simulink model "zengiangcircle"  (Simulink 8.3)
settings: Solver=ode3  StartTime=0.0  StopTime=1500  FixedStep=0.3  RelTol=1e-3
libraries: simulink x1
settings Model: Creator=Administrator  LastModifiedBy=jackyjing
settings OptimizationCC: ExpressionDepthLimit=2147483647
settings DebuggingCC: FcnCallInpInsideContextMsg=UseLocalSettings

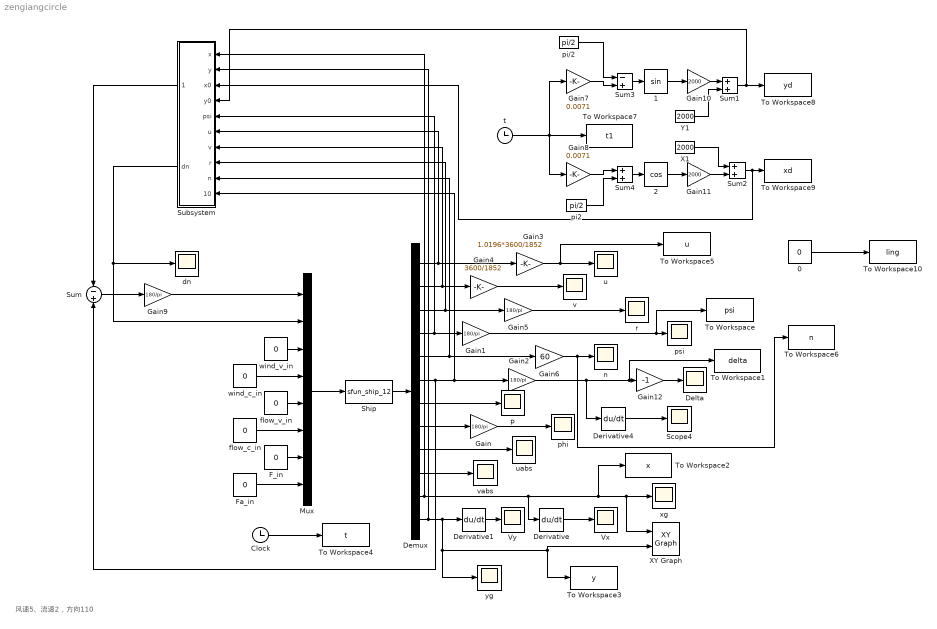
== system zengiangcircle ==
  note: 风速5、流速2，方向110
  "  1" : Trigonometry
  " 2" : Trigonometry  Operator=cos
  0 : Constant  Value=0
  Clock : Clock
  Delta : Scope
      settings: TickLabels=on  TimeRange=1500  YMin=-2  YMax=10  SaveName=ScopeData5
  Demux : Demux  Outputs=12
  Derivative : Derivative
  Derivative1 : Derivative
  Derivative4 : Derivative
  F_in : Constant  Value=0
  Fa_in : Constant  Value=0
  Gain{,1..2,5,9} (5 alike) : Gain  Gain=180/pi
  Gain10 : Gain  Gain=2000
  Gain11 : Gain  Gain=2000
  Gain12 : Gain  Gain=-1
  Gain3 : Gain  Gain=1.0196*3600/1852
  Gain4 : Gain  Gain=3600/1852
  Gain6 : Gain  Gain=60
  Gain7 : Gain  Gain=0.0071
  Gain8 : Gain  Gain=0.0071
  Mux : Mux  Inputs=8
  Scope4 : Scope
      settings: YMin=-0.005  YMax=0.002  SaveName=ScopeData18
  Ship : S-Function  FunctionName=sfun_ship_12  EnableBusSupport=off
  Subsystem : Subsystem
  Sum : Sum  Inputs=-|+
  Sum1 : Sum
  Sum2 : Sum
  Sum3 : Sum  Inputs=-+
  Sum4 : Sum
  To Workspace : ToWorkspace  VariableName=psi  SampleTime=-1
  To Workspace1 : ToWorkspace  VariableName=delta  SampleTime=-1
  To Workspace10 : ToWorkspace  VariableName=ling  SampleTime=-1
  To Workspace2 : ToWorkspace  VariableName=x  SampleTime=-1
  To Workspace3 : ToWorkspace  VariableName=y  SampleTime=-1
  To Workspace4 : ToWorkspace  VariableName=t  SampleTime=-1
  To Workspace5 : ToWorkspace  VariableName=u  SampleTime=-1
  To Workspace6 : ToWorkspace  VariableName=n  SampleTime=-1
  To Workspace7 : ToWorkspace  VariableName=t1  SampleTime=-1
  To Workspace8 : ToWorkspace  VariableName=yd  SampleTime=-1
  To Workspace9 : ToWorkspace  VariableName=xd  SampleTime=-1
  Vx : Scope
      settings: TickLabels=on  SaveName=ScopeData8
  Vy : Scope
      settings: TickLabels=on  SaveName=ScopeData9
  X1 : Constant  Value=2000
  XY Graph : simulink/Sinks/XY Graph  xmin=-1000  xmax=4500  ymin=-1000  ymax=4500  st=-1
  Y1 : Constant  Value=2000
  dn : Scope
      settings: TickLabels=on  YMin=-1.75e-05  YMax=3.75e-05  SaveName=ScopeData21
  flow_c_in : Constant  Value=0
  flow_v_in : Constant  Value=0
  n : Scope
      settings: TickLabels=on  TimeRange=1500  YMin=85.76  YMax=85.97  SaveName=ScopeData4
  p : Scope
      settings: TickLabels=on  SaveName=ScopeData10
  phi : Scope
      settings: YMin=-0.00175  YMax=0.0015  SaveName=ScopeData11
  pi/2 : Constant  Value=pi/2
  "pi2   " : Constant  Value=pi/2
  psi : Scope
      settings: TickLabels=on  TimeRange=500  YMin=-0  YMax=27.5  SaveName=ScopeData3
  r : Scope
      settings: TickLabels=on  SaveName=ScopeData2
  t : Clock
  u : Scope
      settings: TickLabels=on  YMin=25.535  YMax=25.61
  uabs : Scope
      settings: TickLabels=on  YMin=10.75  YMax=15  SaveName=ScopeData6
  v : Scope
      settings: TickLabels=on
  vabs : Scope
      settings: TickLabels=on  YMin=-1.75  YMax=0  SaveName=ScopeData7
  wind_c_in : Constant  Value=0
  wind_v_in : Constant  Value=0
  xg : Scope
      settings: TickLabels=on  YMin=250  YMax=475  SaveName=ScopeData12
  yg : Scope
      settings: TickLabels=on  YMin=250  YMax=475  SaveName=ScopeData13
  wires:
  Ship/1 -> Demux/1
  Demux/1 -> Subsystem/6(u), Gain3/1
  Demux/2 -> Subsystem/7(v), Gain4/1
  Demux/3 -> Subsystem/8(r), Gain5/1
  Demux/5 -> Subsystem/9(n), Gain6/1
  Demux/7 -> p/1
  Demux/8 -> Gain/1
  Gain1/1 -> psi/1, To Workspace/1
  Gain/1 -> phi/1
  Demux/4 -> Subsystem/5(psi), Gain1/1
  Gain3/1 -> To Workspace5/1, u/1
  Gain4/1 -> v/1
  Gain5/1 -> r/1
  Gain6/1 -> To Workspace6/1, n/1
  Demux/9 -> uabs/1
  Demux/10 -> vabs/1
  Demux/12 -> Subsystem/2(y), Derivative1/1, yg/1, To Workspace3/1, XY Graph/2
  Derivative/1 -> Vx/1
  Derivative1/1 -> Vy/1
  wind_v_in/1 -> Mux/3
  wind_c_in/1 -> Mux/4
  flow_v_in/1 -> Mux/5
  F_in/1 -> Mux/7
  Fa_in/1 -> Mux/8
  flow_c_in/1 -> Mux/6
  Mux/1 -> Ship/1
  Derivative4/1 -> Scope4/1
  Clock/1 -> To Workspace4/1
  Sum/1 -> Gain9/1
  Subsystem/1(dpsi) -> Sum/1
  Sum2/1 -> Subsystem/3(x0), To Workspace9/1
  Sum1/1 -> Subsystem/4(y0), To Workspace8/1
  "  1"/1 -> Gain10/1
  " 2"/1 -> Gain11/1
  t/1 -> To Workspace7/1, Gain8/1, Gain7/1
  Gain10/1 -> Sum1/1
  Gain11/1 -> Sum2/2
  X1/1 -> Sum2/1
  Y1/1 -> Sum1/2
  Sum3/1 -> "  1"/1
  Gain7/1 -> Sum3/2
  pi/2/1 -> Sum3/1
  Sum4/1 -> " 2"/1
  Gain8/1 -> Sum4/1
  "pi2   "/1 -> Sum4/2
  Demux/11 -> Subsystem/1(x), Derivative/1, XY Graph/1, xg/1, To Workspace2/1
  Gain9/1 -> Mux/1
  Demux/6 -> Subsystem/10(Delta), Gain2/1, Sum/2
  Subsystem/2(dn) -> dn/1, Mux/2
  0/1 -> To Workspace10/1
  Gain2/1 -> Derivative4/1, To Workspace1/1, Gain12/1
  Gain12/1 -> Delta/1

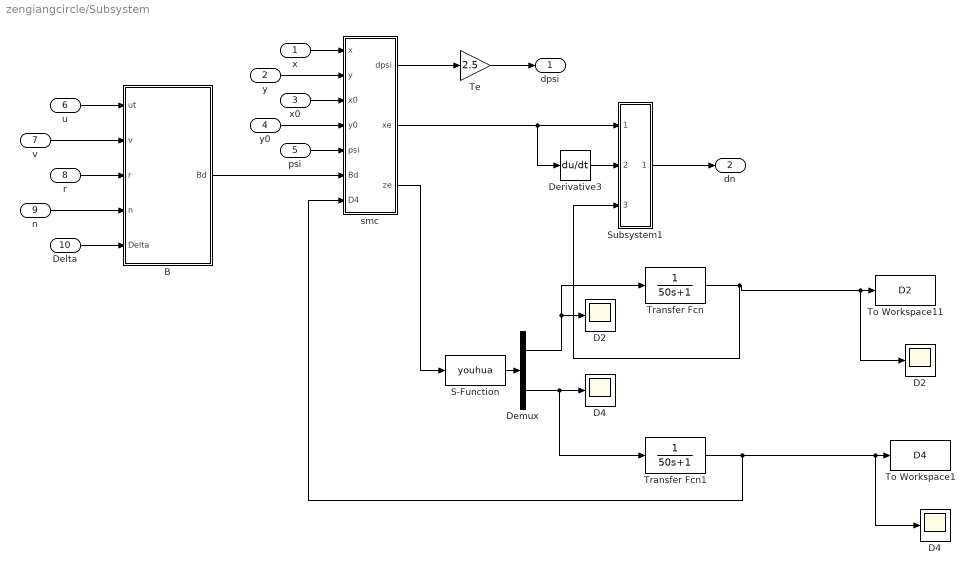
== system zengiangcircle/Subsystem ==
  x : Inport
  y : Inport  Port=2
  x0 : Inport  Port=3
  y0 : Inport  Port=4
  psi : Inport  Port=5
  u : Inport  Port=6
  v : Inport  Port=7
  r : Inport  Port=8
  n : Inport  Port=9
  Delta : Inport  Port=10
  B : MATLAB Function  TreatAsAtomicUnit=on
  D2 : Scope
      settings: TickLabels=on  YMin=1  YMax=11  SaveName=ScopeData22
  "D2 " : Scope
      settings: TickLabels=on  TimeRange=1500  YMin=0.21  YMax=0.41  SaveName=ScopeData24
  D4 : Scope
      settings: TickLabels=on  YMin=500  YMax=1000  SaveName=ScopeData23
  "D4 " : Scope
      settings: TickLabels=on  TimeRange=1500  YMin=747.25  YMax=752  SaveName=ScopeData25
  Demux : Demux  Outputs=2
  Derivative3 : Derivative
  S-Function : S-Function  FunctionName=youhua  EnableBusSupport=off
  Subsystem1 : Subsystem
  Te : Gain  Gain=2.5
  To Workspace1 : ToWorkspace  VariableName=D4  SampleTime=-1
  To Workspace11 : ToWorkspace  VariableName=D2  SampleTime=-1
  Transfer Fcn : TransferFcn  Denominator=[50 1]
  Transfer Fcn1 : TransferFcn  Denominator=[50 1]
  "smc " : Subsystem
  dpsi : Outport
  dn : Outport  Port=2
  wires:
  "smc "/1("dpsi ") -> Te/1
  x/1 -> "smc "/1(x)
  y/1 -> "smc "/2(y)
  x0/1 -> "smc "/3(x0)
  y0/1 -> "smc "/4(y0)
  psi/1 -> "smc "/5("psi ")
  u/1 -> B/1(ut)
  v/1 -> B/2(v)
  r/1 -> B/3(r)
  n/1 -> B/4(n)
  Delta/1 -> B/5(Delta)
  Te/1 -> dpsi/1
  B/1(Bd) -> "smc "/6(Bd)
  Derivative3/1 -> Subsystem1/2(dxe)
  Subsystem1/1(dn) -> dn/1
  "smc "/2(xe) -> Derivative3/1, Subsystem1/1(xe)
  S-Function/1 -> Demux/1
  "smc "/3("ze  ") -> S-Function/1
  Demux/1 -> Transfer Fcn/1, D2/1
  Transfer Fcn/1 -> Subsystem1/3(D2), "D2 "/1, To Workspace11/1
  Demux/2 -> Transfer Fcn1/1, D4/1
  Transfer Fcn1/1 -> "smc "/7(D4), "D4 "/1, To Workspace1/1

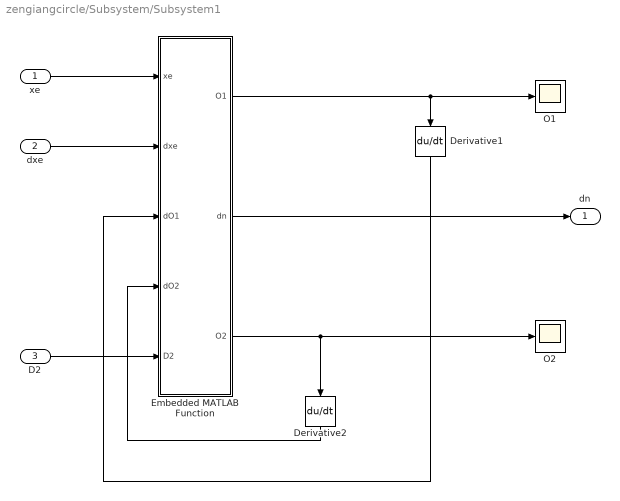
== system zengiangcircle/Subsystem/Subsystem1 ==
  xe : Inport
  dxe : Inport  Port=2
  D2 : Inport  Port=3
  Derivative1 : Derivative
  Derivative2 : Derivative
  Embedded MATLAB Function : MATLAB Function  TreatAsAtomicUnit=on
  O1 : Scope
      settings: TickLabels=on  TimeRange=3000  YMin=-20  YMax=20  SaveName=ScopeData15
  O2 : Scope
      settings: TickLabels=on  TimeRange=3000  YMin=-1  YMax=0.9  SaveName=ScopeData16
  dn : Outport
  wires:
  xe/1 -> Embedded MATLAB Function/1(xe)
  Derivative1/1 -> Embedded MATLAB Function/3(dO1)
  dxe/1 -> Embedded MATLAB Function/2(dxe)
  Derivative2/1 -> Embedded MATLAB Function/4(dO2)
  D2/1 -> Embedded MATLAB Function/5(D2)
  Embedded MATLAB Function/1(O1) -> Derivative1/1, O1/1
  Embedded MATLAB Function/3(O2) -> O2/1, Derivative2/1
  Embedded MATLAB Function/2(dn) -> dn/1

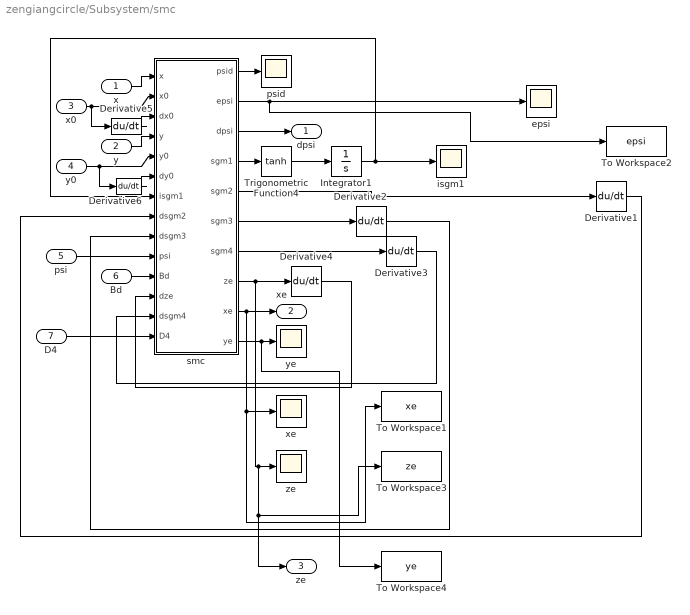
== system zengiangcircle/Subsystem/smc  ==
  x : Inport
  y : Inport  Port=2
  x0 : Inport  Port=3
  y0 : Inport  Port=4
  "psi " : Inport  Port=5
  Bd : Inport  Port=6
  D4 : Inport  Port=7
  Derivative{1..6} (6 alike) : Derivative
  Integrator1 : Integrator
  To Workspace1 : ToWorkspace  VariableName=xe  SampleTime=-1
  To Workspace2 : ToWorkspace  VariableName=epsi  SampleTime=-1
  To Workspace3 : ToWorkspace  VariableName=ze  SampleTime=-1
  To Workspace4 : ToWorkspace  VariableName=ye  SampleTime=-1
  Trigonometric Function4 : Trigonometry  Operator=tanh
  epsi : Scope
      settings: TickLabels=on  YMin=-0.049  YMax=-0.0455  SaveName=ScopeData15
  isgm1 : Scope
      settings: TickLabels=on  YMin=-2200  YMax=0  SaveName=ScopeData16
  psid : Scope
      settings: TickLabels=on  YMin=2.35  YMax=2.7  SaveName=ScopeData17
  "smc " : MATLAB Function  TreatAsAtomicUnit=on
  "xe  " : Scope
      settings: TickLabels=on  YMin=-200  YMax=40  SaveName=ScopeData19
  ye : Scope
      settings: TickLabels=on  YMin=-100  YMax=2000  SaveName=ScopeData14
  "ze " : Scope
      settings: TickLabels=on  TimeRange=1500  YMin=-4.6  YMax=-3.3  SaveName=ScopeData20
  "dpsi " : Outport
  xe : Outport  Port=2
  "ze  " : Outport  Port=3
  wires:
  "smc "/4(sgm1) -> Trigonometric Function4/1
  Derivative2/1 -> "smc "/9(dsgm3)
  Trigonometric Function4/1 -> Integrator1/1
  Derivative1/1 -> "smc "/8(dsgm2)
  x/1 -> "smc "/1(x)
  y/1 -> "smc "/4(y)
  x0/1 -> Derivative5/1, "smc "/2(x0)
  y0/1 -> Derivative6/1, "smc "/5(y0)
  "psi "/1 -> "smc "/10(psi)
  "smc "/3(dpsi) -> "dpsi "/1
  Bd/1 -> "smc "/11(Bd)
  Derivative3/1 -> "smc "/13(dsgm4)
  Derivative4/1 -> "smc "/12(dze)
  "smc "/2(epsi) -> To Workspace2/1, epsi/1
  Integrator1/1 -> "smc "/7(isgm1), isgm1/1
  "smc "/8(ze) -> "ze  "/1, To Workspace3/1, "ze "/1, Derivative4/1
  "smc "/9(xe) -> To Workspace1/1, "xe  "/1, xe/1
  "smc "/10(ye) -> To Workspace4/1, ye/1
  Derivative5/1 -> "smc "/3(dx0)
  Derivative6/1 -> "smc "/6(dy0)
  "smc "/1(psid) -> psid/1
  D4/1 -> "smc "/14(D4)
  "smc "/5(sgm2) -> Derivative1/1
  "smc "/7(sgm4) -> Derivative3/1
  "smc "/6(sgm3) -> Derivative2/1

== matlab function Subsystem/smc /smc  ==
  data: psid output double; epsi output double; x input double; dpsi output double; x0 input double; dx0 input double; y input double; y0 input double; dy0 input double; isgm1 input double; dsgm2 input double; dsgm3 input double; sgm1 output double; sgm2 output double; sgm3 output double; psi input double; Bd input double; dze input double; dsgm4 input double; sgm4 output double; ze output double; xe output double; ye output double; D4 input double
function [psid,epsi,dpsi,sgm1,sgm2,sgm3,sgm4,ze,xe,ye]= fcn(x,x0,dx0,y,y0,dy0,isgm1,dsgm2,dsgm3,psi,Bd,dze,dsgm4,D4)
%#codegen
% k0=0.01;k1=3;k2=0.05;k3=0.005;k4=0.003;k5=0.01;D=200;%ye收敛，xe不收敛
%  k0=0.01;k1=3;k2=0.05;k3=0.05;k4=0.0000003;k5=0.000031;D=200;
%  k0=0.0000001;k1=3;k2=0.00000051;k3=0.1;k4=0.0001;k5=0.00003;D=200;%10.16   k2=0.00000051
% k0=1;k1=3;k2=0.0051;k3=0.1;k4=0.0001;k5=0.00003;D=200;% +|+
 % k0=1;k1=0.03;k2=0.1;k3=0.01;k4=0.001;k5=0.01;D=2;%10.09
%  k0=3;k1=6;k2=0.1;k3=0.01;k4=0.0001;k5=0.03;D=1;%跟踪不上的圆
% k0=1;k1=3;k2=0.0051;k3=0.01;k4=0.01;k5=0.003;D=200;%-|+
% k0=1;k1=3;k2=0.015;k3=0.1;k4=0.00001;k5=0.00003;D=200;% +|+ 10.18
 %  k0=1000;k1=3;k2=0.0005;k3=0.0051;k4=0.06;k5=0.71;D=1;%xe=x-xd,ye=y-yd
% k0=1;k1=3;k2=0.005;k3=0.1;k4=0.00001;k5=0.0045;D=200;%10.19
% k0=0.01;k1=3;k2=0.5;k3=0.1;k4=0.00001;k5=0.01;D=200;
k0=0.01;k1=3;k2=0.05;k3=0.005;k4=0.01;k5=0.01;%10.22   D=200;k5=0.1最好的XY k5=0.2xe最好

% k0=0.01;k1=3;k2=0.05;k3=0.005;k4=0.001;k5=0.001;D=200;


ze=sqrt((x-2000)^2+(y-2000)^2)-2000;
psid=atan2((y-2000),(x-2000));
ye=ze*cos(psid-0.7854)/cos(1.9979);
xe=ze*sin(psid-0.7854)/cos(1.9979);

% psir=atan2(dy0,dx0);
% zitar=atan2((y-y0),(x-x0));
% p=sqrt((x-x0)^2+(y-y0)^2);
% ye=p*sin(zitar-psir);
% xe=p*cos(zitar-psir);


epsi=psi-psid+pi/2;
sgm1=k1*tanh(k0*ze)+dze;
sgm2=epsi+k2*isgm1;
sgm3=k3*tanh(sgm2)+dsgm2;
sgm4=k4*tanh(sgm3)+dsgm3;

dpsi=k5*(1/Bd)*(dsgm4+D4*sgm4);
% dpsi=(1/Bd)*(dsgm4+D*sgm4);

== matlab function Subsystem/B ==
  data: ut input double; Bd output double; v input double; r input double; n input double; Delta input double
function Bd  = fcn(ut,v,r,n,Delta)
% function ud = fcn(ut,v,r,n,Delta,phi,dr,sgm4)
V=sqrt(ut*ut+v*v);%u=x(1) v=x(2)

da=10.5;%9.34+0.25;%尾吃水13.8;%12.5;%
df=7.5;%4.97+0.25;%首吃水14.3;%13.8;%
Dh=9.0;%舵高s   ;%11.411.4;;%+7.00+0.25
pa=1.205;%%%**空气密度
Lpp=267.0;%船长
B=39.8;%船宽
Db=6.466;%舵宽
P=9.657;%da螺距
luow=1026;%小luow是密度 水密度
Dp=9.2;%螺旋桨直径
Ds=23.6;%型深
d=(da+df)/2;%吃水
m=(165.89*d*d + 4383.9*d)*1000;%排水量
Cb=m/(Lpp*B*d*1.025*1000);
AR=(d-7.41)/(12.5-7.41)*(81.44-43.14)+43.14;%舵叶面积
d_B=d/B;L_B=Lpp/B;
mx=m/100*(0.398+11.97*Cb*(1+3.73*d_B)-2.89*Cb*L_B*(1+1.13*d_B)+0.175*Cb*L_B*L_B*(1+0.541*d_B)-1.107*L_B*d_B);
my=m*(0.882-0.54*Cb*(1-1.6*d_B)-0.156*L_B*(1-0.673*Cb)+0.826*d_B*L_B*(1-0.678*d_B)-0.638*Cb*d_B*L_B*(1-0.669*d_B));
wp0=0.5*Cb-0.05;
fa=6.13*Dh/Db/(2.25+Dh/Db);
gma=-22.2*(Cb*B/Lpp)*(Cb*B/Lpp)+0.02*(Cb*B/Lpp)+0.68;
gmaR=1.1633-1.98828*Cb+1.3902*Cb*Cb;
tR=0.7382-0.0539*Cb+0.1755*Cb*Cb;
ifaH=0.6784-1.3374*Cb+1.8891*Cb*Cb;
xH=-(0.4+0.1*Cb)*Lpp;
xR=-0.5*Lpp;
xb=1.87;
Jzz=1/100.0*(33-76.85*Cb*(1-0.784*Cb)+3.43*L_B*(1-0.63*Cb))*Lpp*Lpp;
Izz=(1.0+(Cb^4.5))*m*(Lpp*Lpp+power(B,2.4))/24.0;

m33=Izz+Jzz;

beta=atan2((-v),(ut));%u=x(1) v=x(2)
betap=beta+0.5*r*Lpp/V;%r=x(3)
betaR=beta+r*Lpp/V;
wp=wp0*exp(-4.0*betap*betap);
up=(1.0-wp)*ut;%u=x(1)
s=1.0-up/n/P;% n=x(5)
eta=Dp/Dh;

k=0.6;
Gs=eta*k*(2.0-(2.0-k)*s)*s/(1.0-s)/(1.0-s);
s0=1-(1-wp0)*ut/n/P;% n=x(5)u=x(1)
delt0=-s0/57.3;

if(Delta<0)
    K=1.065;
else
    K=0.935;
end
%
uR=up*(1+K*Gs)^0.5;
vRp=uR*delt0;
vR=vRp-gmaR*(v-Lpp*r);%r=x(3)v=x(2)
UR2=uR*uR+vR*vR;
J=ut*(1-wp)/n/Dp;%u=x(1)  n=x(5)
if(J<=0.3)
    L_ifaH=ifaH*J/0.3;% p137, 3-5-119
else
    L_ifaH=ifaH;
end
%
Bd=(-1.0/2.0)*(xR+L_ifaH*xH)*luow*AR*fa*UR2/(m33);

== matlab function Subsystem/Subsystem1/Embedded MATLAB Function ==
  data: xe input double; dxe input double; dO1 input double; O1 output double; dn output double; dO2 input double; O2 output double; D2 input double
function [O1,dn,O2]=fcn(xe,dxe,dO1,dO2,D2)

% K0=1;K1=1;K2=1;K3=0.01;K4=0.00000001;D=1;%10.09
%K0=1000;K1=1;K2=1;K3=0.01;K4=0.000051;D=1;%10.13
%K0=0.01;K1=1;K2=1;K3=0.1;K4=0.000068;D=1;%卜仁祥
% K0=3;K1=4240;K2=0.00000005;K3=0.01;K4=0.000068;D=1;%K4=0.000068%代昌盛
K0=3;K1=0.0001;K2=0.05;K3=0.05;K4=0.000068;%D=1;
%K0=1;K1=4240;K2=1;K3=0.01;K4=0.0001;D=100;


O1=K1*tanh(K0*xe)+dxe;
O2=K3*tanh(K2*O1)+dO1;
%dn=K4*(1/Bn)*(D*O2+dO2);
dn=K4*(D2*O2+dO2);
